simulink model "Modelo5_2_2"  (R2020a)
settings: Solver=VariableStepAuto  StartTime=0.0  StopTime=50  MaxStep=1e-3  RelTol=1e-3
values from neighbouring files (symbols this model uses):
  alpha_cu = 3.9e-3    (= 0.0039)    [AnalisisDeEstabilidad.m]    (also in LTI_vs_LPV_vs_NL_realimentado.m; Modelo_linealizado.m)
  b_eq = b_m + b_l/(r^2)    (= 2.19444444444e-05)    [LTI_vs_LPV_vs_NL_realimentado.m]    (also in Modelo_linealizado.m)
  ba = 1    [parametros.m]
  C_ts = 0.818    [LTI_vs_LPV_vs_NL_realimentado.m]    (also in Modelo_linealizado.m)
  J_eq = J_m + J_l/(r^2)    (= 1.97847222222e-05)    [LTI_vs_LPV_vs_NL_realimentado.m]    (also in Modelo_linealizado.m)
  Ksa = 1    [parametros.m]
  L_d = 6.6/1000    (= 0.0066)    [Curvas_carc.m]    (also in LTI_vs_LPV_vs_NL_realimentado.m; Modelo_linealizado.m)
  L_ls = 0.8/1000    (= 0.0008)    [LTI_vs_LPV_vs_NL_realimentado.m]    (also in Modelo_linealizado.m)
  L_q = 5.8/1000    (= 0.0058)    [Curvas_carc.m]    (also in LTI_vs_LPV_vs_NL_realimentado.m; Modelo_linealizado.m)
  lambda_m = 0.01546    [Curvas_carc.m]    (also in LTI_vs_LPV_vs_NL_realimentado.m = 0.016; Modelo_linealizado.m = 0.016)
  P_p = 3    [Curvas_carc.m]    (also in LTI_vs_LPV_vs_NL_realimentado.m)
  Pp = 3    [AnalisisDeEstabilidad.m]    (also in LTI_vs_LPV_vs_NL_realimentado.m; Modelo_linealizado.m; parametros.m)
  r = 120    [AnalisisDeEstabilidad.m]    (also in LTI_vs_LPV_vs_NL_realimentado.m; Modelo_linealizado.m; parametros.m)
  R_sREF = R_sref    (= 1.02)    [LTI_vs_LPV_vs_NL_realimentado.m]
  R_ts_amb = 146.7    [LTI_vs_LPV_vs_NL_realimentado.m]    (also in Modelo_linealizado.m)
  Rdp = 3    [parametros.m]
  Rqp = 2    [parametros.m]
  T_sREF = T_sref    (= 40)    [LTI_vs_LPV_vs_NL_realimentado.m]
undefined symbols (not defined in the file or in its folder): K_l, Ksia, R0p, sigbuilder_block
libraries: simulink x3
settings Model: Creator=matie  LastModifiedBy=matie
settings SolverCC: ZeroCrossAlgorithm=Adaptive
settings DebuggingCC: IgnoredZcDiagnostic=none

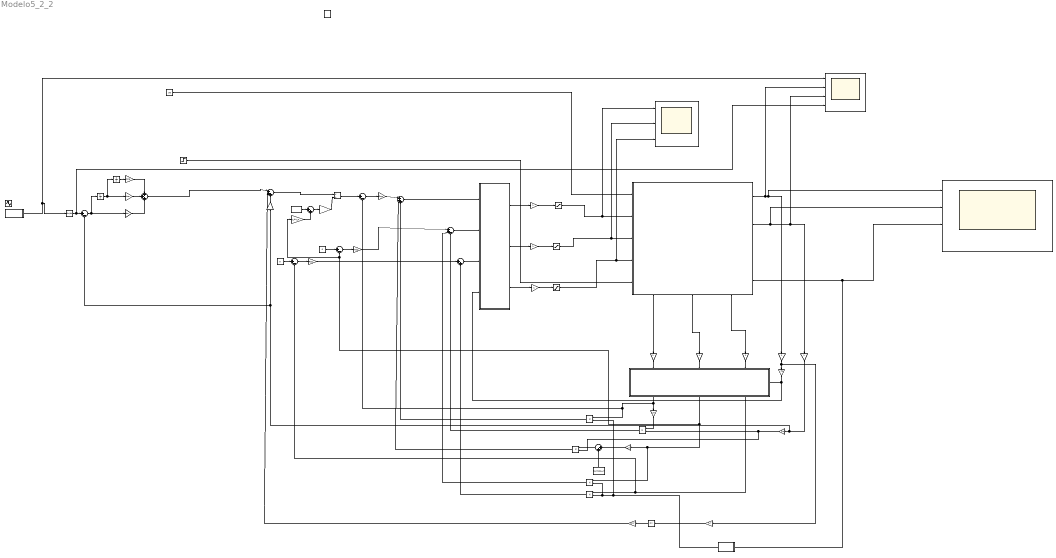
== system Modelo5_2_2 ==
  note: T_m*'
  note: T_m*
  note: V_qs*'
  1/r : Gain  Gain=1/r
  Consigna : Subsystem  Tag=STV Subsys  LoadFcn=sigbuilder_block('load');  StartFcn=sigbuilder_block('start');  StopFcn=sigbuilder_block('stop');  ClipboardFcn=sigbuilder_block('clipboard');  mask(Sigbuilder block){tuvar=[0:10]}
      mask help: Simulink:masks:SigbuilderBlock_MD
      mask init:
      | if ~strcmp(get_param(bdroot(gcbh),'SimulationStatus'),'stopped') tuvar = sigbuilder_block('maskInit'); end
      settings: CopyFcn=sigbuilder_block('copy');  DeleteFcn=sigbuilder_block('delete');  ModelCloseFcn=sigbuilder_block('modelClose');  PreSaveFcn=sigbuilder_block('preSave');  PauseFcn=sigbuilder_block('pause');  ContinueFcn=sigbuilder_block('continue');  NameChangeFcn=sigbuilder_block('namechange');  OpenFcn=sigbuilder_block('open',[6 30 837.75 681.75 ]);  CloseFcn=sigbuilder_block('close');
      mask Display: plot(0, 0, 100, 100,[2, 2, 32, 32, 2], [68, 8, 8, 68, 68],[32, 2], [38, 38], [32, 19, 2],[53, 60, 44], [32, 17, 17, 2],[16, 16, 31, 31]);txt = getActiveGroup(gcbh);text(2, 100, txt,'verticalAlignment', 'top');
  Constant1 : Constant  Value=0
  Constant2 : Constant  Value=lambda_m
  Constant3 : Constant  Value=0
  Constant4 : Constant  Value=lambda_m
  Derivative : Derivative  CoefficientInTFapproximation=0
  Divide : Product  Inputs=*/
  Evolución R_s : Subsystem
  Gain1 : Gain  Gain=Ksia
  Gain11 : Gain  Gain=R0p
  Gain12 : Gain  Gain=Ksa
  Gain13 : Gain  Gain=ba
  Gain3 : Gain  Gain=b_eq
  Gain4 : Gain  Gain=L_d-L_q
  Gain5 : Gain  Gain=3*P_p/2
  Gain6 : Gain  Gain=Rqp
  Gain8 : Gain  Gain=Rdp
  Int1 : Integrator
  Int2 : Integrator
  Inv_a : Gain
  Inv_b : Gain
  Inv_c : Gain
  Kl/r : Gain  Gain=K_l/r
  Ld1 : Gain  Gain=L_d
  Lq1 : Gain  Gain=L_q
  Planta : Subsystem
      settings: PortSchema="{\"entries\":[{\"content\":{\"sides\":[{\"content\":{\"connectorIds\":[\"In1\",\"In2\",\"In3\",\"In4\",\"In5\"]},\"type\":\"ConnectorPlacement.EquallySpacedRectSide\",\"uuid\":\"7dd159b7-6d73-44ef-8a17-1619ab3a0fe8\"},{\"content\":{\"connectorIds\":[\"Out1\",\"Out2\",\"Out3\",\"Out4\"],\"side\":\"RIGHT\"},\"type\":\"ConnectorPlacement.EquallySpacedRectSide\",\"uuid\":\"f05f5aa2-2d36-48ca-b041-91fd4aa476a9\"},{\"content\":{\"connectorIds\":[],\"side\":\"TOP\"},\"type\":\"ConnectorPlacement.EquallySpacedRectSide\",\"uuid\":\"f00a682c-ef39-4c36-94cc-25936eb5c6a2\"},{\"content\":{\"connectorIds\":[\"Out5\",\"Out6\",\"Out7\"],\"side\":\"BOTTOM\"},\"type\":\"ConnectorPlacement.EquallySpacedRectSide\",\"uuid\":\"801a9ef0-d698-4696-ba24-5671b76f5cda\"}]},\"type\":\"ConnectorPlacement.EquallySpacedConnector\",\"uuid\":\"0722cfee-bb25-4366-9e08-c5916c966df5\"}],\"packageUris\":[\"http://schema.mathworks.com/mf0/Connector/19700101\"],\"version\":\"1.0\"}"
  Pp2 : Gain  Gain=Pp
  Pp3 : Gain  Gain=Pp
  Product{,1..4} (5 alike) : Product
  Saturation : Saturate  UpperLimit=20  LowerLimit=-20
  Saturation1 : Saturate  UpperLimit=20  LowerLimit=-20
  Saturation2 : Saturate  UpperLimit=20  LowerLimit=-20
  Scope : Scope  NumInputPorts=4
  Scope1 : Scope  NumInputPorts=4
  Scope2 : Scope  NumInputPorts=3
  Sen_Pos : Gain
  Sen_Vel : Gain
  Sen_a : Gain
  Sen_b : Gain
  Sen_c : Gain
  Sine Wave : Sin  Amplitude=50  Frequency=2*pi/5  SampleTime=0
  Step : Step  Time=15  After=7  SampleTime=0
  Sum{10,13,15,29} (4 alike) : Sum  Inputs=|+-
  Sum11 : Sum  Inputs=|+++
  Sum12 : Sum  Inputs=|++
  Sum14 : Sum  Inputs=+++
  Sum28 : Sum  Inputs=|++
  Sum7 : Sum  Inputs=|++-
  Sum8 : Sum  Inputs=|+++
  Sum9 : Sum  Inputs=|++
  T.Park1 : Subsystem
      settings: PortSchema="{\"entries\":[{\"content\":{\"sides\":[{\"content\":{\"connectorIds\":[\"In1\",\"In2\",\"In3\"]},\"type\":\"ConnectorPlacement.EquallySpacedRectSide\",\"uuid\":\"2bfbe7ef-652a-4797-b13c-b84c243bd68c\"},{\"content\":{\"connectorIds\":[\"Out1\",\"Out2\",\"Out3\"],\"side\":\"RIGHT\"},\"type\":\"ConnectorPlacement.EquallySpacedRectSide\",\"uuid\":\"075def0e-c436-44dc-ba25-82cf6ffae869\"},{\"content\":{\"connectorIds\":[],\"side\":\"TOP\"},\"type\":\"ConnectorPlacement.EquallySpacedRectSide\",\"uuid\":\"95d81334-e332-4f04-a2cb-c4692f91809c\"},{\"content\":{\"connectorIds\":[\"In4\"],\"side\":\"BOTTOM\"},\"type\":\"ConnectorPlacement.EquallySpacedRectSide\",\"uuid\":\"85b95360-e43d-49d1-a18f-690334b045e6\"}]},\"type\":\"ConnectorPlacement.EquallySpacedConnector\",\"uuid\":\"b90f9cad-0277-459c-bcac-17172872a787\"}],\"packageUris\":[\"http://schema.mathworks.com/mf0/Connector/19700101\"],\"version\":\"1.0\"}"
  T.ParkInv1 : Subsystem
  TempAmb : Constant  Value=30
  Trigonometric Function2 : Trigonometry
  XY Graph : simulink/Sinks/XY Graph  IOType=viewer  xmin=-1  xmax=1  ymin=-1  ymax=1  st=-1
  XY Graph1 : simulink/Sinks/XY Graph  IOType=viewer  xmin=-1  xmax=1  ymin=-1  ymax=1  st=-1
  wires:
  Lq1/1 -> Product3/1
  Planta/5(I_a) -> Sen_a/1  "Ia"
  Pp2/1 -> Product4/2, Product3/2
  Product3/1 -> Sum7/3  "Vd*"
  T.Park1/1(q) -> Product2/1, Sum10/2, Lq1/1  "iq"
  Planta/7(I_c) -> Sen_c/1  "Ic"
  T.ParkInv1/3(c) -> Inv_c/1  "Vc"
  Planta/6(I_b) -> Sen_b/1  "Ib"
  T.ParkInv1/2(b) -> Inv_b/1  "Vb"
  Sen_c/1 -> T.Park1/3(c)
  Sen_b/1 -> T.Park1/2(b)
  Sen_a/1 -> T.Park1/1(a)
  T.ParkInv1/1(a) -> Inv_a/1  "Va"
  Sen_Pos/1 -> 1/r/1, Pp3/1
  Sum7/1 -> T.ParkInv1/2(d)
  Constant2/1 -> Sum9/2
  Ld1/1 -> Sum9/1
  Sum9/1 -> Product4/1
  T.Park1/2(d) -> Gain4/1, Sum13/2, Product1/1, Ld1/1  "id"
  Product4/1 -> Sum8/2
  Sum8/1 -> T.ParkInv1/1(q)
  Sum11/1 -> Divide/1
  Sen_Vel/1 -> Pp2/1, Sum15/2, Gain3/1
  Sum12/1 -> Gain5/1
  Gain5/1 -> Divide/2
  Gain4/1 -> Sum12/2
  Gain3/1 -> Sum11/3
  Constant4/1 -> Sum12/1
  Product2/1 -> Sum8/3
  Sum10/1 -> Gain6/1
  Divide/1 -> Sum10/1  "I_qs*"
  Gain6/1 -> Sum8/1
  Product1/1 -> Sum7/2
  Sum13/1 -> Gain8/1
  Constant1/1 -> Sum13/1
  Gain8/1 -> Sum7/1
  Sum28/1 -> T.ParkInv1/3(0)
  Product/1 -> Sum28/2
  Sum29/1 -> Gain11/1
  T.Park1/3(0) -> Product/1, Sum29/2  "i0"
  Constant3/1 -> Sum29/1
  Gain11/1 -> Sum28/1
  Trigonometric Function2/1 -> Kl/r/1
  Pp3/1 -> T.ParkInv1/4(Pos. Electrica), T.Park1/4(Pos. Electrica)
  1/r/1 -> Trigonometric Function2/1
  Inv_c/1 -> Saturation2/1
  Inv_b/1 -> Saturation1/1
  Inv_a/1 -> Saturation/1
  Planta/1(theta_m) -> Scope1/2, Scope/1, Sen_Pos/1  "Pos_m2"
  Planta/2(omega_m) -> Scope/2, Scope1/3, Sen_Vel/1  "Vel_m2"
  Planta/4(T_s) -> Evolución R_s/1(T_s), Scope/3  "Ts2"
  TempAmb/1 -> Planta/1(T_amb)
  Step/1 -> Planta/5(T_d)  "Td"
  Evolución R_s/1(R_s) -> Product2/2, Product1/2, Product/2
  Gain1/1 -> Sum14/1
  Gain13/1 -> Sum14/3
  Int1/1 -> Gain1/1
  Sum15/1 -> Int2/1, Gain13/1
  Gain12/1 -> Sum14/2
  Int2/1 -> Gain12/1, Int1/1
  Derivative/1 -> Scope1/4, Sum15/1  "omega_m*"
  Sum14/1 -> Sum11/1
  Kl/r/1 -> Sum11/2
  Consigna/1(Signal 1) -> Scope1/1, Derivative/1
  Saturation/1 -> Scope2/1, Planta/2(V_a)
  Saturation1/1 -> Scope2/2, Planta/3(V_b)
  Saturation2/1 -> Scope2/3, Planta/4(V_c)

== system Modelo5_2_2/Consigna ==
  Demux : Demux  Tag=STV Demux  Outputs=1
      settings: DisplayOption=none
  FromWs : FromWorkspace  Tag=STV FromWs  VariableName=tuvar
      SigBuilderData=|
      | common.afterFinalStr = 'Extrapolate'
      | common.sampleTime = 0
      | dataSet.timeRange = [0 10]
      | dataSet.name = 'Group 1'
      | sbobj.Groups.Name = 'Group 1'
      | sbobj.Groups.Signals.Name = 'Signal 1'
      | sbobj.Groups.Signals.XData = [0 0.3 1 2 3 5 7 10]
      | sbobj.Groups.Signals.YData = [0 0 6.28 6.28 -6.28 -6.28 0 0]
  Signal 1 : Outport  Tag=STV Outport
  wires:
  Demux/1 -> Signal 1/1
  FromWs/1 -> Demux/1

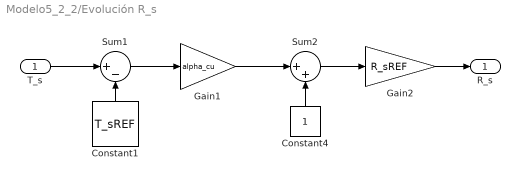
== system Modelo5_2_2/Evolución R_s ==
  T_s : Inport
  Constant1 : Constant  Value=T_sREF
  Constant4 : Constant
  Gain1 : Gain  Gain=alpha_cu
  Gain2 : Gain  Gain=R_sREF
  Sum1 : Sum  Inputs=|+-
  Sum2 : Sum  Inputs=|++
  R_s : Outport
  wires:
  Sum2/1 -> Gain2/1
  Constant4/1 -> Sum2/2
  T_s/1 -> Sum1/1
  Sum1/1 -> Gain1/1
  Gain1/1 -> Sum2/1
  Constant1/1 -> Sum1/2
  Gain2/1 -> R_s/1

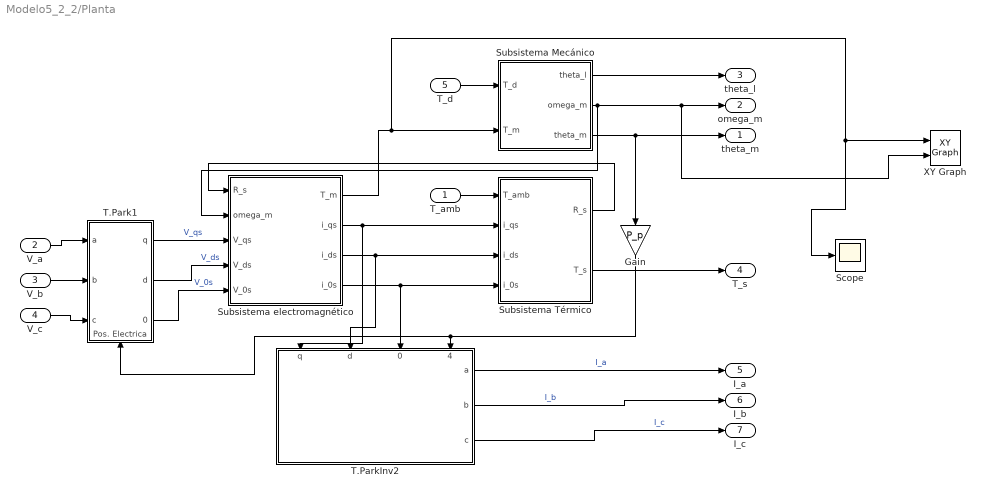
== system Modelo5_2_2/Planta ==
  T_amb : Inport
  V_a : Inport  Port=2
  V_b : Inport  Port=3
  V_c : Inport  Port=4
  T_d : Inport  Port=5
  "\tSubsistema Térmico" : Subsystem
  Gain : Gain  Gain=P_p
  Scope : Scope
  Subsistema Mecánico : Subsystem
  Subsistema electromagnético : Subsystem
  T.Park1 : Subsystem
      settings: PortSchema="{\"entries\":[{\"content\":{\"sides\":[{\"content\":{\"connectorIds\":[\"In1\",\"In2\",\"In3\"]},\"type\":\"ConnectorPlacement.EquallySpacedRectSide\",\"uuid\":\"2bfbe7ef-652a-4797-b13c-b84c243bd68c\"},{\"content\":{\"connectorIds\":[\"Out1\",\"Out2\",\"Out3\"],\"side\":\"RIGHT\"},\"type\":\"ConnectorPlacement.EquallySpacedRectSide\",\"uuid\":\"075def0e-c436-44dc-ba25-82cf6ffae869\"},{\"content\":{\"connectorIds\":[\"In4\"],\"side\":\"TOP\"},\"type\":\"ConnectorPlacement.EquallySpacedRectSide\",\"uuid\":\"95d81334-e332-4f04-a2cb-c4692f91809c\"},{\"content\":{\"connectorIds\":[],\"side\":\"BOTTOM\"},\"type\":\"ConnectorPlacement.EquallySpacedRectSide\",\"uuid\":\"85b95360-e43d-49d1-a18f-690334b045e6\"}]},\"type\":\"ConnectorPlacement.EquallySpacedConnector\",\"uuid\":\"b90f9cad-0277-459c-bcac-17172872a787\"}],\"packageUris\":[\"http://schema.mathworks.com/mf0/Connector/19700101\"],\"version\":\"1.0\"}"
  T.ParkInv2 : Subsystem
      settings: PortSchema="{\"entries\":[{\"content\":{\"sides\":[{\"content\":{\"connectorIds\":[\"In1\",\"In2\",\"In3\",\"In4\"]},\"type\":\"ConnectorPlacement.EquallySpacedRectSide\",\"uuid\":\"afd1bd75-d36d-487c-add7-d7d974f3fb5b\"},{\"content\":{\"connectorIds\":[],\"side\":\"RIGHT\"},\"type\":\"ConnectorPlacement.EquallySpacedRectSide\",\"uuid\":\"1b08b6e4-620f-4af3-9003-41050c957193\"},{\"content\":{\"connectorIds\":[],\"side\":\"TOP\"},\"type\":\"ConnectorPlacement.EquallySpacedRectSide\",\"uuid\":\"b726a9b4-8f78-46b8-a7b9-dcfad0016e42\"},{\"content\":{\"connectorIds\":[\"Out1\",\"Out2\",\"Out3\"],\"side\":\"BOTTOM\"},\"type\":\"ConnectorPlacement.EquallySpacedRectSide\",\"uuid\":\"1b0b5e0b-11cb-4e38-80d3-f3707e0a92c3\"}]},\"type\":\"ConnectorPlacement.EquallySpacedConnector\",\"uuid\":\"8a718423-2b24-4423-b930-b070c3f08686\"}],\"packageUris\":[\"http://schema.mathworks.com/mf0/Connector/19700101\"],\"version\":\"1.0\"}"
  XY Graph : simulink/Sinks/XY Graph  xmin=-3  xmax=3  ymin=-100  ymax=500  st=-1
  theta_m : Outport
  omega_m : Outport  Port=2
  theta_l : Outport  Port=3
  T_s : Outport  Port=4
  I_a : Outport  Port=5
  I_b : Outport  Port=6
  I_c : Outport  Port=7
  wires:
  Subsistema Mecánico/3(theta_m) -> Gain/1, theta_m/1
  Gain/1 -> T.Park1/4(Pos. Electrica), T.ParkInv2/4(Pos. Electrica)
  T.Park1/3(q) -> Subsistema electromagnético/3(V_qs)  "V_qs"
  Subsistema Mecánico/2(omega_m) -> Subsistema electromagnético/2(omega_m), XY Graph/2, omega_m/1
  Subsistema electromagnético/2(i_qs) -> "\tSubsistema Térmico"/2(i_qs), T.ParkInv2/1(q)
  Subsistema electromagnético/1(T_m) -> Scope/1, XY Graph/1, Subsistema Mecánico/2(T_m)
  Subsistema electromagnético/4(i_0s) -> "\tSubsistema Térmico"/4(i_0s), T.ParkInv2/3(0)
  V_c/1 -> T.Park1/1(c)
  T.ParkInv2/3(c) -> I_c/1  "I_c"
  T.ParkInv2/2(b) -> I_b/1  "I_b"
  Subsistema electromagnético/3(i_ds) -> "\tSubsistema Térmico"/3(i_ds), T.ParkInv2/2(d)
  V_b/1 -> T.Park1/2(b)
  Subsistema Mecánico/1(theta_l) -> theta_l/1
  T.ParkInv2/1(a) -> I_a/1  "I_a"
  T.Park1/1(0) -> Subsistema electromagnético/5(V_0s)  "V_0s"
  V_a/1 -> T.Park1/3(a)
  T.Park1/2(d) -> Subsistema electromagnético/4(V_ds)  "V_ds"
  T_d/1 -> Subsistema Mecánico/1(T_d)
  T_amb/1 -> "\tSubsistema Térmico"/1(T_amb)
  "\tSubsistema Térmico"/1(R_s) -> Subsistema electromagnético/1(R_s)
  "\tSubsistema Térmico"/2(T_s) -> T_s/1

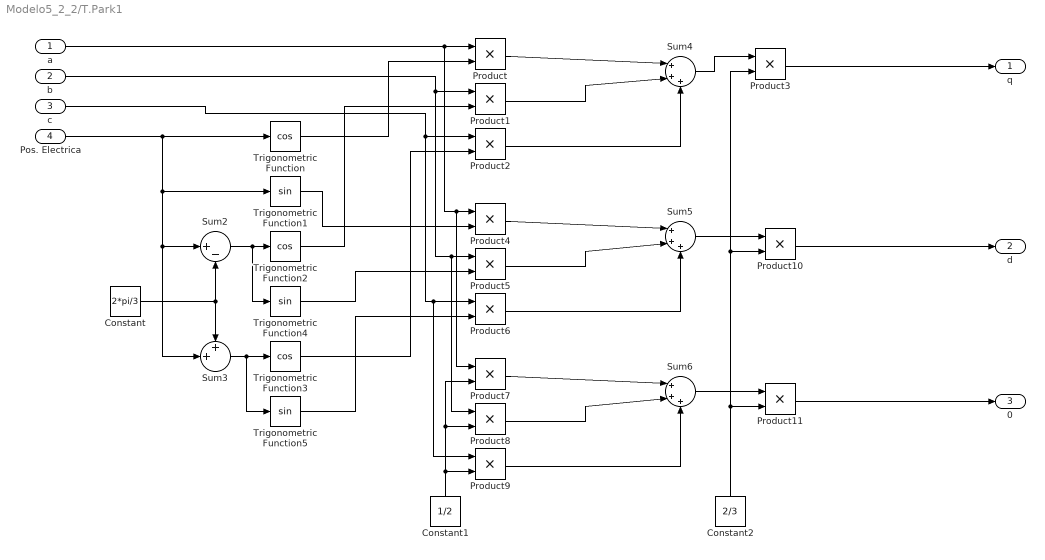
== system Modelo5_2_2/T.Park1 ==
  a : Inport
  b : Inport  Port=2
  c : Inport  Port=3
  Pos. Electrica : Inport  Port=4
  Constant : Constant  Value=2*pi/3
  Constant1 : Constant  Value=1/2
  Constant2 : Constant  Value=2/3
  Product{,1..11} (12 alike) : Product
  Sum2 : Sum  Inputs=|+-
  Sum3 : Sum  Inputs=++|
  Sum4 : Sum  Inputs=|+++
  Sum5 : Sum  Inputs=|+++
  Sum6 : Sum  Inputs=|+++
  Trigonometric Function : Trigonometry  Operator=cos
  Trigonometric Function1 : Trigonometry
  Trigonometric Function2 : Trigonometry  Operator=cos
  Trigonometric Function3 : Trigonometry  Operator=cos
  Trigonometric Function4 : Trigonometry
  Trigonometric Function5 : Trigonometry
  q : Outport
  d : Outport  Port=2
  0 : Outport  Port=3
  wires:
  Product1/1 -> Sum4/2
  c/1 -> Product9/1, Product6/1, Product2/1
  Constant1/1 -> Product9/2, Product8/2, Product7/2
  Sum2/1 -> Trigonometric Function4/1, Trigonometric Function2/1
  Constant2/1 -> Product11/2, Product10/2, Product3/2
  b/1 -> Product8/1, Product5/1, Product1/1
  Product11/1 -> 0/1
  Pos. Electrica/1 -> Sum3/2, Sum2/1, Trigonometric Function1/1, Trigonometric Function/1
  Trigonometric Function2/1 -> Product1/2
  Trigonometric Function5/1 -> Product6/2
  Product6/1 -> Sum5/3
  Trigonometric Function1/1 -> Product4/2
  Constant/1 -> Sum3/1, Sum2/2
  Sum5/1 -> Product10/1
  Product3/1 -> q/1
  Sum4/1 -> Product3/1
  Trigonometric Function3/1 -> Product2/2
  Trigonometric Function/1 -> Product/2
  a/1 -> Product7/1, Product4/1, Product/1
  Product10/1 -> d/1
  Trigonometric Function4/1 -> Product5/2
  Product/1 -> Sum4/1
  Product7/1 -> Sum6/1
  Sum3/1 -> Trigonometric Function5/1, Trigonometric Function3/1
  Product2/1 -> Sum4/3
  Product9/1 -> Sum6/3
  Product5/1 -> Sum5/2
  Product4/1 -> Sum5/1
  Sum6/1 -> Product11/1
  Product8/1 -> Sum6/2

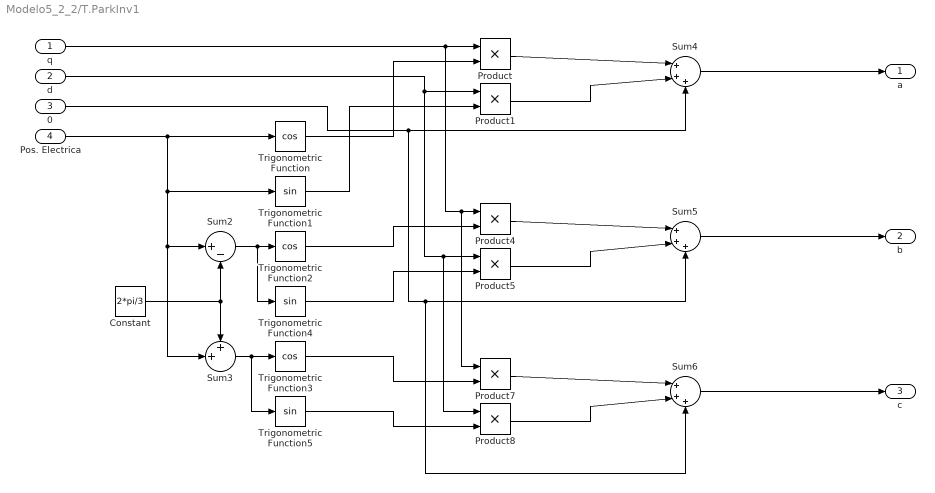
== system Modelo5_2_2/T.ParkInv1 ==
  q : Inport
  d : Inport  Port=2
  0 : Inport  Port=3
  Pos. Electrica : Inport  Port=4
  Constant : Constant  Value=2*pi/3
  Product{,1,4..5,7..8} (6 alike) : Product
  Sum2 : Sum  Inputs=|+-
  Sum3 : Sum  Inputs=++|
  Sum4 : Sum  Inputs=|+++
  Sum5 : Sum  Inputs=|+++
  Sum6 : Sum  Inputs=|+++
  Trigonometric Function : Trigonometry  Operator=cos
  Trigonometric Function1 : Trigonometry
  Trigonometric Function2 : Trigonometry  Operator=cos
  Trigonometric Function3 : Trigonometry  Operator=cos
  Trigonometric Function4 : Trigonometry
  Trigonometric Function5 : Trigonometry
  a : Outport
  b : Outport  Port=2
  c : Outport  Port=3
  wires:
  Constant/1 -> Sum3/1, Sum2/2
  Pos. Electrica/1 -> Sum3/2, Sum2/1, Trigonometric Function1/1, Trigonometric Function/1
  Trigonometric Function3/1 -> Product7/2
  d/1 -> Product8/1, Product5/1, Product1/1
  0/1 -> Sum4/3, Sum5/3, Sum6/3
  Product8/1 -> Sum6/2
  Product7/1 -> Sum6/1
  q/1 -> Product7/1, Product4/1, Product/1
  Sum3/1 -> Trigonometric Function5/1, Trigonometric Function3/1
  Trigonometric Function5/1 -> Product8/2
  Sum6/1 -> c/1
  Product1/1 -> Sum4/2
  Sum2/1 -> Trigonometric Function4/1, Trigonometric Function2/1
  Sum4/1 -> a/1
  Sum5/1 -> b/1
  Trigonometric Function1/1 -> Product1/2
  Product5/1 -> Sum5/2
  Trigonometric Function2/1 -> Product4/2
  Product4/1 -> Sum5/1
  Product/1 -> Sum4/1
  Trigonometric Function/1 -> Product/2
  Trigonometric Function4/1 -> Product5/2

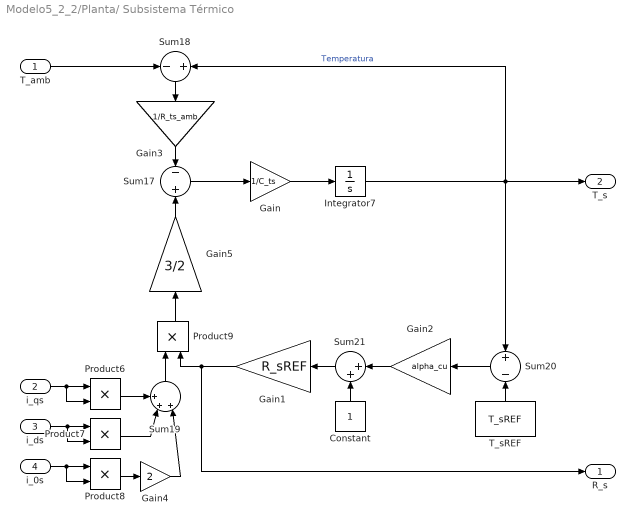
== system Modelo5_2_2/Planta/	Subsistema Térmico ==
  T_amb : Inport
  i_qs : Inport  Port=2
  i_ds : Inport  Port=3
  i_0s : Inport  Port=4
  Constant : Constant
  Gain : Gain  Gain=1/C_ts
  Gain1 : Gain  Gain=R_sREF
  Gain2 : Gain  Gain=alpha_cu
  Gain3 : Gain  Gain=1/R_ts_amb
  Gain4 : Gain  Gain=2
  Gain5 : Gain  Gain=3/2
  Integrator7 : Integrator  InitialCondition=25
  Product{6..9} (4 alike) : Product
  Sum17 : Sum  Inputs=-+
  Sum18 : Sum  Inputs=-+
  Sum19 : Sum  Inputs=+++|
  Sum20 : Sum  Inputs=+-
  Sum21 : Sum  Inputs=|++
  T_sREF : Constant  Value=T_sREF
  R_s : Outport
  T_s : Outport  Port=2
  wires:
  Gain4/1 -> Sum19/3
  Integrator7/1 -> Sum18/2, T_s/1, Sum20/1  "Temperatura"
  Sum21/1 -> Gain1/1
  i_ds/1 -> Product7/2, Product7/1
  Product8/1 -> Gain4/1
  Product7/1 -> Sum19/2
  T_amb/1 -> Sum18/1
  Sum18/1 -> Gain3/1
  Product6/1 -> Sum19/1
  Gain/1 -> Integrator7/1
  Product9/1 -> Gain5/1
  Sum17/1 -> Gain/1
  Gain3/1 -> Sum17/1
  T_sREF/1 -> Sum20/2
  Sum20/1 -> Gain2/1
  Gain1/1 -> Product9/2, R_s/1
  i_qs/1 -> Product6/1, Product6/2
  Sum19/1 -> Product9/1
  Gain2/1 -> Sum21/1
  i_0s/1 -> Product8/2, Product8/1
  Constant/1 -> Sum21/2
  Gain5/1 -> Sum17/2

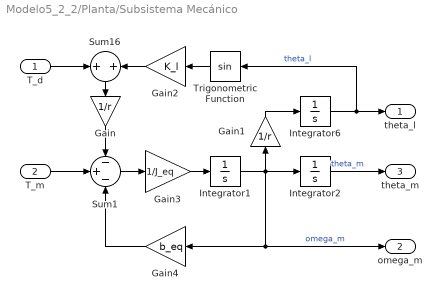
== system Modelo5_2_2/Planta/Subsistema Mecánico ==
  T_d : Inport
  T_m : Inport  Port=2
  Gain : Gain  Gain=1/r
  Gain1 : Gain  Gain=1/r
  Gain2 : Gain  Gain=K_l
  Gain3 : Gain  Gain=1/J_eq
  Gain4 : Gain  Gain=b_eq
  Integrator1 : Integrator
  Integrator2 : Integrator
  Integrator6 : Integrator
  Sum1 : Sum  Inputs=-+-
  Sum16 : Sum  Inputs=+|+
  Trigonometric Function : Trigonometry
  theta_l : Outport
  omega_m : Outport  Port=2
  theta_m : Outport  Port=3
  wires:
  Integrator2/1 -> theta_m/1  "theta_m"
  Integrator6/1 -> theta_l/1, Trigonometric Function/1  "theta_l"
  Gain1/1 -> Integrator6/1
  Gain4/1 -> Sum1/3
  T_m/1 -> Sum1/2
  Integrator1/1 -> Gain4/1, omega_m/1, Integrator2/1, Gain1/1  "omega_m"
  Trigonometric Function/1 -> Gain2/1
  Gain2/1 -> Sum16/2
  Sum16/1 -> Gain/1
  Gain/1 -> Sum1/1
  T_d/1 -> Sum16/1
  Sum1/1 -> Gain3/1
  Gain3/1 -> Integrator1/1

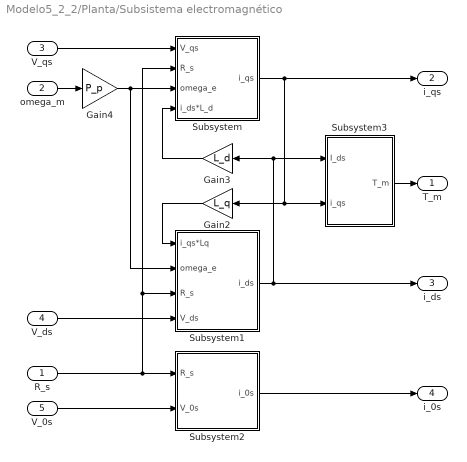
== system Modelo5_2_2/Planta/Subsistema electromagnético ==
  R_s : Inport
  omega_m : Inport  Port=2
  V_qs : Inport  Port=3
  V_ds : Inport  Port=4
  V_0s : Inport  Port=5
  Gain2 : Gain  Gain=L_q
  Gain3 : Gain  Gain=L_d
  Gain4 : Gain  Gain=P_p
  Subsystem : Subsystem
  Subsystem1 : Subsystem
  Subsystem2 : Subsystem
  Subsystem3 : Subsystem
  T_m : Outport
  i_qs : Outport  Port=2
  i_ds : Outport  Port=3
  i_0s : Outport  Port=4
  wires:
  omega_m/1 -> Gain4/1
  Subsystem/1(i_qs) -> i_qs/1, Subsystem3/2(i_qs), Gain2/1
  Subsystem1/1(i_ds) -> i_ds/1, Subsystem3/1(I_ds), Gain3/1
  Gain2/1 -> Subsystem1/1(i_qs*Lq)
  Gain3/1 -> Subsystem/4(i_ds*L_d)
  Gain4/1 -> Subsystem1/2(omega_e), Subsystem/3(omega_e)
  V_qs/1 -> Subsystem/1(V_qs)
  R_s/1 -> Subsystem/2(R_s), Subsystem1/3(R_s), Subsystem2/1(R_s)
  V_ds/1 -> Subsystem1/4(V_ds)
  V_0s/1 -> Subsystem2/2(V_0s)
  Subsystem2/1(i_0s) -> i_0s/1
  Subsystem3/1(T_m) -> T_m/1

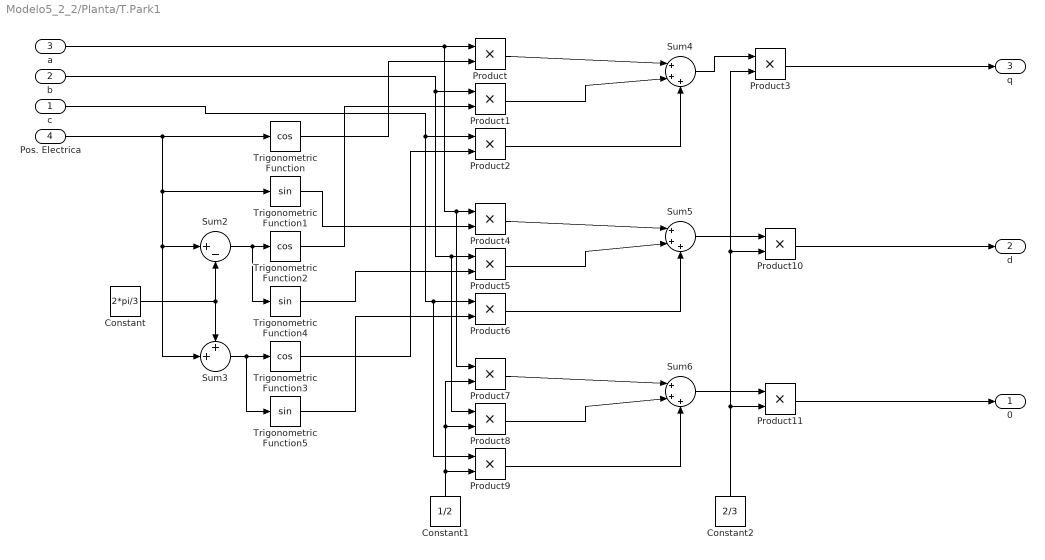
== system Modelo5_2_2/Planta/T.Park1 ==
  c : Inport
  b : Inport  Port=2
  a : Inport  Port=3
  Pos. Electrica : Inport  Port=4
  Constant : Constant  Value=2*pi/3
  Constant1 : Constant  Value=1/2
  Constant2 : Constant  Value=2/3
  Product{,1..11} (12 alike) : Product
  Sum2 : Sum  Inputs=|+-
  Sum3 : Sum  Inputs=++|
  Sum4 : Sum  Inputs=|+++
  Sum5 : Sum  Inputs=|+++
  Sum6 : Sum  Inputs=|+++
  Trigonometric Function : Trigonometry  Operator=cos
  Trigonometric Function1 : Trigonometry
  Trigonometric Function2 : Trigonometry  Operator=cos
  Trigonometric Function3 : Trigonometry  Operator=cos
  Trigonometric Function4 : Trigonometry
  Trigonometric Function5 : Trigonometry
  0 : Outport
  d : Outport  Port=2
  q : Outport  Port=3
  wires:
  Product1/1 -> Sum4/2
  c/1 -> Product9/1, Product6/1, Product2/1
  Constant1/1 -> Product9/2, Product8/2, Product7/2
  Sum2/1 -> Trigonometric Function4/1, Trigonometric Function2/1
  Constant2/1 -> Product11/2, Product10/2, Product3/2
  b/1 -> Product8/1, Product5/1, Product1/1
  Product11/1 -> 0/1
  Pos. Electrica/1 -> Sum3/2, Sum2/1, Trigonometric Function1/1, Trigonometric Function/1
  Trigonometric Function2/1 -> Product1/2
  Trigonometric Function5/1 -> Product6/2
  Product6/1 -> Sum5/3
  Trigonometric Function1/1 -> Product4/2
  Constant/1 -> Sum3/1, Sum2/2
  Sum5/1 -> Product10/1
  Product3/1 -> q/1
  Sum4/1 -> Product3/1
  Trigonometric Function3/1 -> Product2/2
  Trigonometric Function/1 -> Product/2
  a/1 -> Product7/1, Product4/1, Product/1
  Product10/1 -> d/1
  Trigonometric Function4/1 -> Product5/2
  Product/1 -> Sum4/1
  Product7/1 -> Sum6/1
  Sum3/1 -> Trigonometric Function5/1, Trigonometric Function3/1
  Product2/1 -> Sum4/3
  Product9/1 -> Sum6/3
  Product5/1 -> Sum5/2
  Product4/1 -> Sum5/1
  Sum6/1 -> Product11/1
  Product8/1 -> Sum6/2

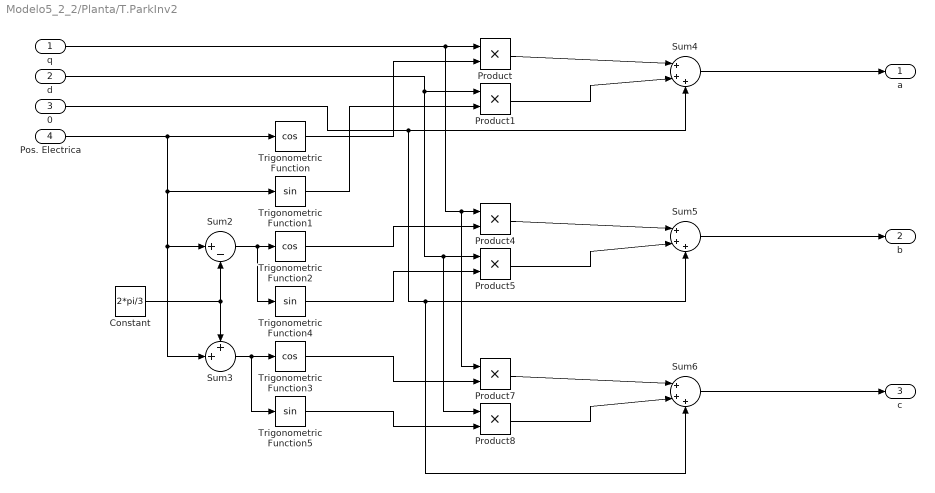
== system Modelo5_2_2/Planta/T.ParkInv2 ==
  q : Inport
  d : Inport  Port=2
  0 : Inport  Port=3
  Pos. Electrica : Inport  Port=4
  Constant : Constant  Value=2*pi/3
  Product{,1,4..5,7..8} (6 alike) : Product
  Sum2 : Sum  Inputs=|+-
  Sum3 : Sum  Inputs=++|
  Sum4 : Sum  Inputs=|+++
  Sum5 : Sum  Inputs=|+++
  Sum6 : Sum  Inputs=|+++
  Trigonometric Function : Trigonometry  Operator=cos
  Trigonometric Function1 : Trigonometry
  Trigonometric Function2 : Trigonometry  Operator=cos
  Trigonometric Function3 : Trigonometry  Operator=cos
  Trigonometric Function4 : Trigonometry
  Trigonometric Function5 : Trigonometry
  a : Outport
  b : Outport  Port=2
  c : Outport  Port=3
  wires:
  Constant/1 -> Sum3/1, Sum2/2
  Pos. Electrica/1 -> Sum3/2, Sum2/1, Trigonometric Function1/1, Trigonometric Function/1
  Trigonometric Function3/1 -> Product7/2
  d/1 -> Product8/1, Product5/1, Product1/1
  0/1 -> Sum4/3, Sum5/3, Sum6/3
  Product8/1 -> Sum6/2
  Product7/1 -> Sum6/1
  q/1 -> Product7/1, Product4/1, Product/1
  Sum3/1 -> Trigonometric Function5/1, Trigonometric Function3/1
  Trigonometric Function5/1 -> Product8/2
  Sum6/1 -> c/1
  Product1/1 -> Sum4/2
  Sum2/1 -> Trigonometric Function4/1, Trigonometric Function2/1
  Sum4/1 -> a/1
  Sum5/1 -> b/1
  Trigonometric Function1/1 -> Product1/2
  Product5/1 -> Sum5/2
  Trigonometric Function2/1 -> Product4/2
  Product4/1 -> Sum5/1
  Product/1 -> Sum4/1
  Trigonometric Function/1 -> Product/2
  Trigonometric Function4/1 -> Product5/2

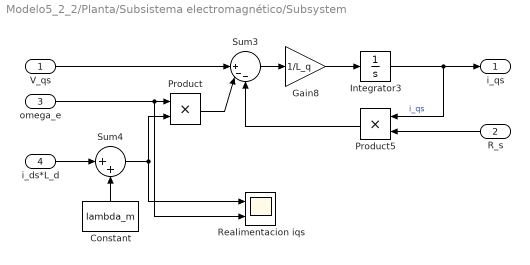
== system Modelo5_2_2/Planta/Subsistema electromagnético/Subsystem ==
  V_qs : Inport
  R_s : Inport  Port=2
  omega_e : Inport  Port=3
  i_ds*L_d : Inport  Port=4
  Constant : Constant  Value=lambda_m
  Gain8 : Gain  Gain=1/L_q
  Integrator3 : Integrator
  Product : Product
  Product5 : Product
  Realimentacion iqs : Scope  NumInputPorts=2
  Sum3 : Sum  Inputs=||+--
  Sum4 : Sum  Inputs=|++
  i_qs : Outport
  wires:
  Constant/1 -> Sum4/2
  Product5/1 -> Sum3/3
  V_qs/1 -> Sum3/1
  i_ds*L_d/1 -> Sum4/1
  Product/1 -> Sum3/2
  Gain8/1 -> Integrator3/1
  Integrator3/1 -> Product5/1, i_qs/1  "i_qs"
  Sum4/1 -> Product/2, Realimentacion iqs/1
  Sum3/1 -> Gain8/1
  R_s/1 -> Product5/2
  omega_e/1 -> Realimentacion iqs/2, Product/1

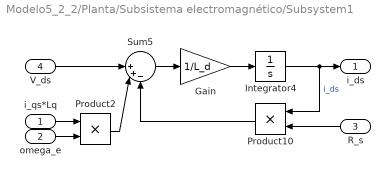
== system Modelo5_2_2/Planta/Subsistema electromagnético/Subsystem1 ==
  i_qs*Lq : Inport
  omega_e : Inport  Port=2
  R_s : Inport  Port=3
  V_ds : Inport  Port=4
  Gain : Gain  Gain=1/L_d
  Integrator4 : Integrator
  Product10 : Product
  Product2 : Product
  Sum5 : Sum  Inputs=||++-
  i_ds : Outport
  wires:
  Product10/1 -> Sum5/3
  i_qs*Lq/1 -> Product2/1
  Gain/1 -> Integrator4/1
  V_ds/1 -> Sum5/1
  Sum5/1 -> Gain/1
  R_s/1 -> Product10/2
  Product2/1 -> Sum5/2
  omega_e/1 -> Product2/2
  Integrator4/1 -> i_ds/1, Product10/1  "i_ds"

== system Modelo5_2_2/Planta/Subsistema electromagnético/Subsystem2 ==
  R_s : Inport
  V_0s : Inport  Port=2
  Gain1 : Gain  Gain=1/L_ls
  Integrator5 : Integrator
  Product11 : Product
  Sum6 : Sum  Inputs=|+-
  i_0s : Outport
  wires:
  Integrator5/1 -> i_0s/1, Product11/1  "i_0s"
  Product11/1 -> Sum6/2
  R_s/1 -> Product11/2
  Sum6/1 -> Gain1/1
  Gain1/1 -> Integrator5/1
  V_0s/1 -> Sum6/1

== system Modelo5_2_2/Planta/Subsistema electromagnético/Subsystem3 ==
  I_ds : Inport
  i_qs : Inport  Port=2
  Gain5 : Gain  Gain=L_d-L_q
  Gain6 : Gain  Gain=3*P_p/2
  Gain7 : Gain  Gain=lambda_m
  Product1 : Product
  Sum2 : Sum  Inputs=|++
  T_m : Outport
  wires:
  Sum2/1 -> Gain6/1
  Gain7/1 -> Sum2/1
  I_ds/1 -> Product1/2
  Gain5/1 -> Sum2/2
  i_qs/1 -> Product1/1, Gain7/1
  Gain6/1 -> T_m/1
  Product1/1 -> Gain5/1
